simulink subsystem "Battery_Model"  (R2022a)
settings: Solver=VariableStepAuto  StartTime=0.0  StopTime=10.0  RelTol=1e-3
undefined symbols (not defined in the file): Battery, Np_Module
libraries: fl_lib x580, nesl_utility x386, ee_lib x96, simulink x96
(part 1 of 6)
settings Model: Creator=The MathWorks, Inc.  LastModifiedBy=The MathWorks, Inc.
settings SolverCC: MaxZcPerStep=1
settings DebuggingCC: UnconnectedInputMsg=warning  UnconnectedOutputMsg=warning  UnconnectedLineMsg=warning
settings RTWCC: DLArmComputeVersion=19.05

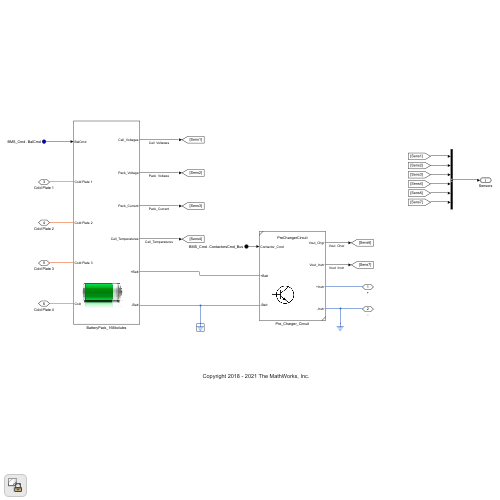
[thumbnail: Simulink's stored preview of the top-level diagram]
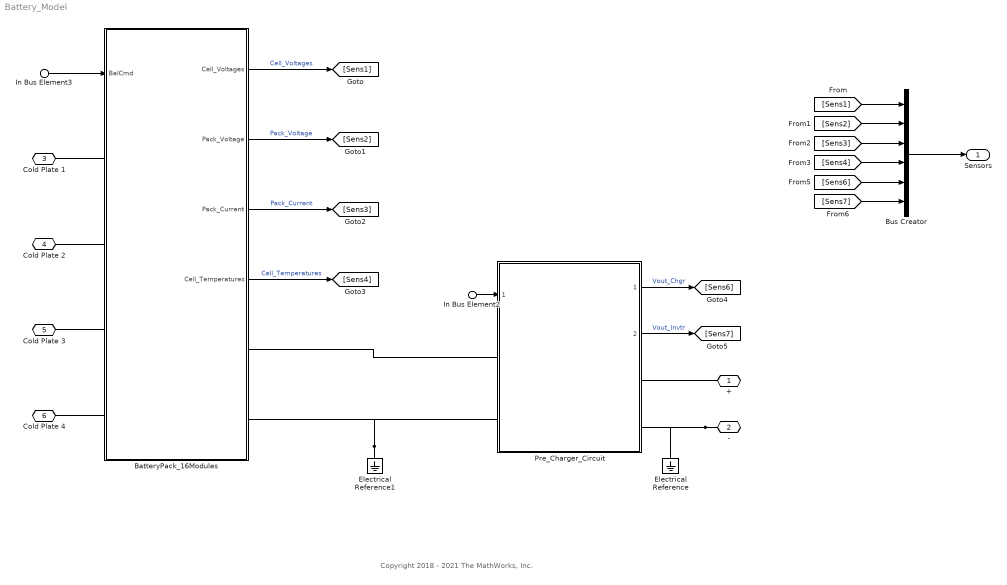
== system Battery_Model ==
  note: Copyright 2018 - 2021 The MathWorks, Inc.
  In Bus Element2 : Inport  PortName=BMS_Cmd  Element=ContactorsCmd_Bus
  In Bus Element3 : Inport  PortName=BMS_Cmd  Element=BalCmd
  BatteryPack_16Modules : Subsystem  VariantControl=NumModules == 16
      mask Display: image('Plant_Battery.jpg',[20,45,120,70])
  Bus Creator : BusCreator  Inputs=6  OutDataTypeStr=Bus: Sensors  NonVirtualBus=on
      settings: InheritFromInputs=off
  Electrical Reference : fl_lib/Electrical/Electrical Elements/Electrical Reference
      settings: SourceProductBaseCode=PW,SS,VE
  Electrical Reference1 : fl_lib/Electrical/Electrical Elements/Electrical Reference
      settings: SourceProductBaseCode=PW,SS,VE
  Pre_Charger_Circuit : Subsystem  ReferencedSubsystem=PreChangerCircuit
  + : PMIOPort  Side=Right
  - : PMIOPort  Port=2  Side=Right
  Cold Plate 1 : PMIOPort  Port=3  Side=Left
  Cold Plate 2 : PMIOPort  Port=4  Side=Left
  Cold Plate 3 : PMIOPort  Port=5  Side=Left
  Cold Plate 4 : PMIOPort  Port=6  Side=Left
  Sensors : Outport  OutDataTypeStr=Bus: Sensors  VectorParamsAs1DForOutWhenUnconnected=off  BusOutputAsStruct=on
  wires:
  [Sens6] -> Bus Creator/5
  Pre_Charger_Circuit/1 -> [Sens6]  "Vout_Chgr"
  [Sens3] -> Bus Creator/3
  In Bus Element2/1 -> Pre_Charger_Circuit/1
  [Sens7] -> Bus Creator/6
  [Sens1] -> Bus Creator/1
  [Sens2] -> Bus Creator/2
  [Sens4] -> Bus Creator/4
  Pre_Charger_Circuit/2 -> [Sens7]  "Vout_Invtr"
  BatteryPack_16Modules/1(Cell_Voltages) -> [Sens1]  "Cell_Voltages"
  Bus Creator/1 -> Sensors/1
  BatteryPack_16Modules/4(Cell_Temperatures) -> [Sens4]  "Cell_Temperatures"
  BatteryPack_16Modules/3(Pack_Current) -> [Sens3]  "Pack_Current"
  BatteryPack_16Modules/2(Pack_Voltage) -> [Sens2]  "Pack_Voltage"
  In Bus Element3/1 -> BatteryPack_16Modules/1(BalCmd)
  connections:
  -/RConn1 -- Electrical Reference/LConn1 -- Pre_Charger_Circuit/RConn2
  Electrical Reference1/LConn1 -- BatteryPack_16Modules/RConn2 -- Pre_Charger_Circuit/LConn2
  Pre_Charger_Circuit/RConn1 -- +/RConn1
  Pre_Charger_Circuit/LConn1 -- BatteryPack_16Modules/RConn1
  Cold Plate 1/RConn1 -- BatteryPack_16Modules/LConn1
  Cold Plate 2/RConn1 -- BatteryPack_16Modules/LConn2
  Cold Plate 3/RConn1 -- BatteryPack_16Modules/LConn3
  Cold Plate 4/RConn1 -- BatteryPack_16Modules/LConn4

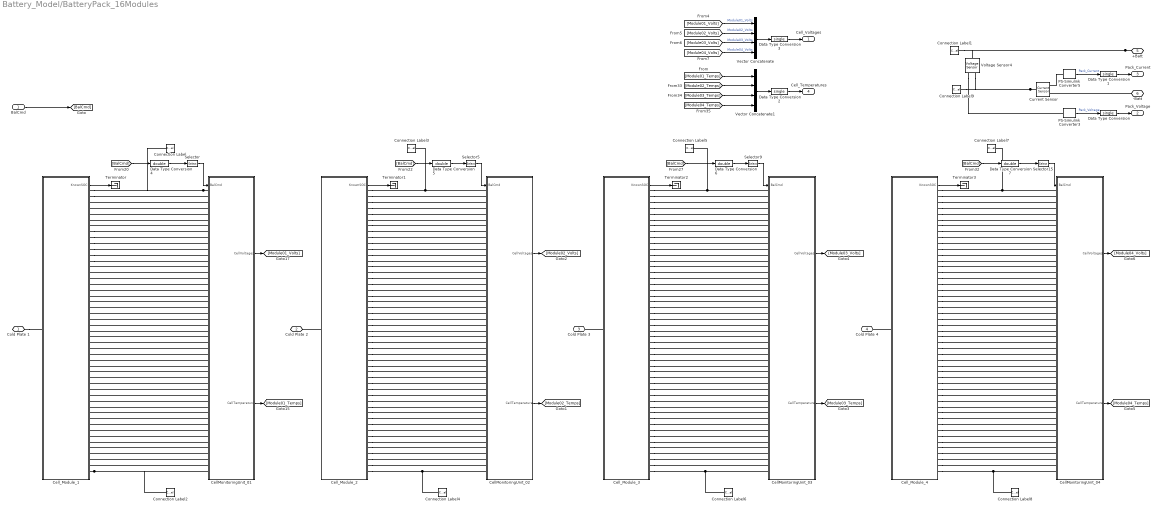
== system Battery_Model/BatteryPack_16Modules ==
  BalCmd : Inport
  CellMonitoringUnit_01 : Subsystem
  CellMonitoringUnit_02 : Subsystem
  CellMonitoringUnit_03 : Subsystem
  CellMonitoringUnit_04 : Subsystem
  Cell_Module_1 : Subsystem
  Cell_Module_2 : Subsystem
  Cell_Module_3 : Subsystem
  Cell_Module_4 : Subsystem
  Connection Label : ConnectionLabel  Label=BattPos
  Connection Label1 : ConnectionLabel  Label=BattPos
  Connection Label2 : ConnectionLabel  Label=BattA
  Connection Label3 : ConnectionLabel  Label=BattA
  Connection Label4 : ConnectionLabel  Label=BattB
  Connection Label5 : ConnectionLabel  Label=BattB
  Connection Label6 : ConnectionLabel  Label=BattC
  Connection Label7 : ConnectionLabel  Label=BattC
  Connection Label8 : ConnectionLabel  Label=BattNeg
  Connection Label9 : ConnectionLabel  Label=BattNeg
  Current Sensor : fl_lib/Electrical/Electrical Sensors/Current Sensor
      settings: SourceProductBaseCode=PW,SS,VE
  Data Type Conversion{,1..3} (4 alike) : DataTypeConversion  OutDataTypeStr=single  SaturateOnIntegerOverflow=off  RndMeth=Floor
  Data Type Conversion{4..7} (4 alike) : DataTypeConversion  OutDataTypeStr=double  SaturateOnIntegerOverflow=off  RndMeth=Floor
  PS-Simulink Converter3 : nesl_utility/PS-Simulink Converter  PhysicalDomain=network_engine_domain  SubClassName=ps_output  LeftPortType=input  RightPortType=output  PseudoPeriodic=off  Frequencies=[]  VectorFormat=1-D array  Unit=V  AffineConversion=off
      settings: SourceProductBaseCode=SS,PW,VE
  PS-Simulink Converter5 : nesl_utility/PS-Simulink Converter  PhysicalDomain=network_engine_domain  SubClassName=ps_output  LeftPortType=input  RightPortType=output  PseudoPeriodic=off  Frequencies=[]  VectorFormat=1-D array  Unit=A  AffineConversion=off
      settings: SourceProductBaseCode=SS,PW,VE
  Selector : Selector  InputPortWidth=96  IndexOptions=Starting index (dialog)  Indices=[1]  OutputSizes=24
  Selector15 : Selector  InputPortWidth=96  IndexOptions=Starting index (dialog)  Indices=73  OutputSizes=24
  Selector5 : Selector  InputPortWidth=96  IndexOptions=Starting index (dialog)  Indices=25  OutputSizes=24
  Selector9 : Selector  InputPortWidth=96  IndexOptions=Starting index (dialog)  Indices=49  OutputSizes=24
  Terminator{,1..3} (4 alike) : Terminator
  Vector Concatenate : Concatenate  NumInputs=4
  Vector Concatenate1 : Concatenate  NumInputs=4
  Voltage Sensor4 : fl_lib/Electrical/Electrical Sensors/Voltage Sensor
      settings: SourceProductBaseCode=PW,SS,VE
  Cold Plate 1 : PMIOPort  Side=Left
  Cold Plate 2 : PMIOPort  Port=2  Side=Left
  Cold Plate 3 : PMIOPort  Port=3  Side=Left
  Cold Plate 4 : PMIOPort  Port=4  Side=Left
  +Batt : PMIOPort  Port=5  Side=Right
  -Batt : PMIOPort  Port=6  Side=Right
  Cell_Voltages : Outport  VectorParamsAs1DForOutWhenUnconnected=off
  Pack_Voltage : Outport  Port=2  VectorParamsAs1DForOutWhenUnconnected=off
  Pack_Current : Outport  Port=3  VectorParamsAs1DForOutWhenUnconnected=off
  Cell_Temperatures : Outport  Port=4  VectorParamsAs1DForOutWhenUnconnected=off
  wires:
  Data Type Conversion7/1 -> Selector15/1
  Data Type Conversion6/1 -> Selector9/1
  Data Type Conversion5/1 -> Selector5/1
  Data Type Conversion4/1 -> Selector/1
  CellMonitoringUnit_04/2(CellTemperature) -> [Module04_Temps]
  Cell_Module_4/1(KnownSOC) -> Terminator3/1
  CellMonitoringUnit_04/1(CellVoltages) -> [Module04_Volts]
  Selector15/1 -> CellMonitoringUnit_04/1(BalCmd)
  CellMonitoringUnit_03/2(CellTemperature) -> [Module03_Temps]
  Cell_Module_3/1(KnownSOC) -> Terminator2/1
  CellMonitoringUnit_03/1(CellVoltages) -> [Module03_Volts]
  Selector9/1 -> CellMonitoringUnit_03/1(BalCmd)
  CellMonitoringUnit_02/2(CellTemperature) -> [Module02_Temps]
  Cell_Module_2/1(KnownSOC) -> Terminator1/1
  CellMonitoringUnit_02/1(CellVoltages) -> [Module02_Volts]
  Selector5/1 -> CellMonitoringUnit_02/1(BalCmd)
  Cell_Module_1/1(KnownSOC) -> Terminator/1
  Data Type Conversion3/1 -> Cell_Voltages/1
  Data Type Conversion2/1 -> Cell_Temperatures/1
  CellMonitoringUnit_01/1(CellVoltages) -> [Module01_Volts]
  CellMonitoringUnit_01/2(CellTemperature) -> [Module01_Temps]
  Vector Concatenate1/1 -> Data Type Conversion2/1
  [Module04_Temps] -> Vector Concatenate1/4
  [Module03_Temps] -> Vector Concatenate1/3
  [Module02_Temps] -> Vector Concatenate1/2
  [Module01_Temps] -> Vector Concatenate1/1
  Data Type Conversion1/1 -> Pack_Current/1
  Data Type Conversion/1 -> Pack_Voltage/1
  [BalCmd] -> Data Type Conversion7/1
  [BalCmd] -> Data Type Conversion6/1
  [BalCmd] -> Data Type Conversion5/1
  Selector/1 -> CellMonitoringUnit_01/1(BalCmd)
  [BalCmd] -> Data Type Conversion4/1
  [Module04_Volts] -> Vector Concatenate/4  "Module04_Volts"
  [Module03_Volts] -> Vector Concatenate/3  "Module03_Volts"
  [Module02_Volts] -> Vector Concatenate/2  "Module02_Volts"
  Vector Concatenate/1 -> Data Type Conversion3/1
  [Module01_Volts] -> Vector Concatenate/1  "Module01_Volts"
  PS-Simulink Converter5/1 -> Data Type Conversion1/1  "Pack_Current"
  PS-Simulink Converter3/1 -> Data Type Conversion/1  "Pack_Voltage"
  BalCmd/1 -> [BalCmd]
  connections:
  Cell_Module_4/RConn40 -- CellMonitoringUnit_04/LConn40
  Cell_Module_4/RConn10 -- CellMonitoringUnit_04/LConn10
  Cell_Module_4/RConn35 -- CellMonitoringUnit_04/LConn35
  Cell_Module_4/RConn24 -- CellMonitoringUnit_04/LConn24
  Cell_Module_4/RConn5 -- CellMonitoringUnit_04/LConn5
  Cell_Module_4/RConn44 -- CellMonitoringUnit_04/LConn44
  Cell_Module_4/RConn29 -- CellMonitoringUnit_04/LConn29
  Cell_Module_4/RConn33 -- CellMonitoringUnit_04/LConn33
  Cell_Module_4/RConn3 -- CellMonitoringUnit_04/LConn3
  Cell_Module_4/RConn9 -- CellMonitoringUnit_04/LConn9
  Cell_Module_4/RConn30 -- CellMonitoringUnit_04/LConn30
  Cell_Module_4/RConn18 -- CellMonitoringUnit_04/LConn18
  Cell_Module_4/RConn16 -- CellMonitoringUnit_04/LConn16
  Cell_Module_4/RConn19 -- CellMonitoringUnit_04/LConn19
  Cell_Module_4/RConn36 -- CellMonitoringUnit_04/LConn36
  Cell_Module_4/RConn46 -- CellMonitoringUnit_04/LConn46
  Cell_Module_4/RConn4 -- CellMonitoringUnit_04/LConn4
  Cell_Module_4/RConn47 -- CellMonitoringUnit_04/LConn47
  Cell_Module_4/RConn20 -- CellMonitoringUnit_04/LConn20
  Cell_Module_4/RConn42 -- CellMonitoringUnit_04/LConn42
  Cell_Module_4/RConn27 -- CellMonitoringUnit_04/LConn27
  Cell_Module_4/RConn32 -- CellMonitoringUnit_04/LConn32
  Cell_Module_4/RConn23 -- CellMonitoringUnit_04/LConn23
  Cell_Module_4/RConn15 -- CellMonitoringUnit_04/LConn15
  Cell_Module_4/RConn45 -- CellMonitoringUnit_04/LConn45
  Cell_Module_4/RConn17 -- CellMonitoringUnit_04/LConn17
  Cell_Module_4/RConn39 -- CellMonitoringUnit_04/LConn39
  Cell_Module_4/RConn12 -- CellMonitoringUnit_04/LConn12
  Cell_Module_4/RConn26 -- CellMonitoringUnit_04/LConn26
  Cell_Module_4/RConn6 -- CellMonitoringUnit_04/LConn6
  Cell_Module_4/RConn21 -- CellMonitoringUnit_04/LConn21
  Cell_Module_4/RConn48 -- CellMonitoringUnit_04/LConn48
  Cell_Module_4/RConn2 -- CellMonitoringUnit_04/LConn2
  Cell_Module_4/RConn31 -- CellMonitoringUnit_04/LConn31
  Cell_Module_4/RConn11 -- CellMonitoringUnit_04/LConn11
  Cell_Module_4/RConn38 -- CellMonitoringUnit_04/LConn38
  Cell_Module_4/RConn14 -- CellMonitoringUnit_04/LConn14
  Cell_Module_4/RConn8 -- CellMonitoringUnit_04/LConn8
  Cell_Module_4/RConn22 -- CellMonitoringUnit_04/LConn22
  Cell_Module_4/RConn13 -- CellMonitoringUnit_04/LConn13
  Cell_Module_4/RConn34 -- CellMonitoringUnit_04/LConn34
  Cell_Module_4/LConn1 -- Cold Plate 4/RConn1
  Cell_Module_4/RConn37 -- CellMonitoringUnit_04/LConn37
  Cell_Module_4/RConn43 -- CellMonitoringUnit_04/LConn43
  Cell_Module_4/RConn41 -- CellMonitoringUnit_04/LConn41
  Cell_Module_4/RConn7 -- CellMonitoringUnit_04/LConn7
  Cell_Module_4/RConn28 -- CellMonitoringUnit_04/LConn28
  Cell_Module_4/RConn25 -- CellMonitoringUnit_04/LConn25
  Cell_Module_4/RConn49 -- Connection Label8/LConn1 -- CellMonitoringUnit_04/LConn49
  Cell_Module_4/RConn1 -- Connection Label7/LConn1 -- CellMonitoringUnit_04/LConn1
  Cell_Module_3/RConn18 -- CellMonitoringUnit_03/LConn18
  Cell_Module_3/RConn10 -- CellMonitoringUnit_03/LConn10
  Cell_Module_3/RConn39 -- CellMonitoringUnit_03/LConn39
  Cell_Module_3/RConn44 -- CellMonitoringUnit_03/LConn44
  Cell_Module_3/RConn46 -- CellMonitoringUnit_03/LConn46
  Cell_Module_3/RConn24 -- CellMonitoringUnit_03/LConn24
  Cell_Module_3/RConn33 -- CellMonitoringUnit_03/LConn33
  Cell_Module_3/RConn32 -- CellMonitoringUnit_03/LConn32
  Cell_Module_3/RConn5 -- CellMonitoringUnit_03/LConn5
  Cell_Module_3/RConn17 -- CellMonitoringUnit_03/LConn17
  Cell_Module_3/RConn29 -- CellMonitoringUnit_03/LConn29
  Cell_Module_3/RConn9 -- CellMonitoringUnit_03/LConn9
  Cell_Module_3/RConn16 -- CellMonitoringUnit_03/LConn16
  Cell_Module_3/RConn48 -- CellMonitoringUnit_03/LConn48
  Cell_Module_3/RConn19 -- CellMonitoringUnit_03/LConn19
  Cell_Module_3/RConn36 -- CellMonitoringUnit_03/LConn36
  Cell_Module_3/RConn11 -- CellMonitoringUnit_03/LConn11
  Cell_Module_3/RConn4 -- CellMonitoringUnit_03/LConn4
  Cell_Module_3/RConn47 -- CellMonitoringUnit_03/LConn47
  Cell_Module_3/RConn20 -- CellMonitoringUnit_03/LConn20
  Cell_Module_3/RConn42 -- CellMonitoringUnit_03/LConn42
  Cell_Module_3/RConn21 -- CellMonitoringUnit_03/LConn21
  Cell_Module_3/RConn45 -- CellMonitoringUnit_03/LConn45
  Cell_Module_3/RConn15 -- CellMonitoringUnit_03/LConn15
  Cell_Module_3/RConn30 -- CellMonitoringUnit_03/LConn30
  Cell_Module_3/RConn31 -- CellMonitoringUnit_03/LConn31
  Cell_Module_3/RConn23 -- CellMonitoringUnit_03/LConn23
  Cell_Module_3/RConn40 -- CellMonitoringUnit_03/LConn40
  Cell_Module_3/RConn35 -- CellMonitoringUnit_03/LConn35
  Cell_Module_3/RConn12 -- CellMonitoringUnit_03/LConn12
  Cell_Module_3/RConn26 -- CellMonitoringUnit_03/LConn26
  Cell_Module_3/RConn6 -- CellMonitoringUnit_03/LConn6
  Cell_Module_3/RConn2 -- CellMonitoringUnit_03/LConn2
  Cell_Module_3/RConn38 -- CellMonitoringUnit_03/LConn38
  Cell_Module_3/RConn3 -- CellMonitoringUnit_03/LConn3
  Cell_Module_3/RConn8 -- CellMonitoringUnit_03/LConn8
  Cell_Module_3/RConn25 -- CellMonitoringUnit_03/LConn25
  Cell_Module_3/RConn22 -- CellMonitoringUnit_03/LConn22
  Cell_Module_3/RConn13 -- CellMonitoringUnit_03/LConn13
  Cell_Module_3/RConn14 -- CellMonitoringUnit_03/LConn14
  Cell_Module_3/RConn34 -- CellMonitoringUnit_03/LConn34
  Cell_Module_3/RConn37 -- CellMonitoringUnit_03/LConn37
  Cell_Module_3/RConn43 -- CellMonitoringUnit_03/LConn43
  Cell_Module_3/RConn41 -- CellMonitoringUnit_03/LConn41
  Cell_Module_3/LConn1 -- Cold Plate 3/RConn1
  Cell_Module_3/RConn7 -- CellMonitoringUnit_03/LConn7
  Cell_Module_3/RConn28 -- CellMonitoringUnit_03/LConn28
  Cell_Module_3/RConn27 -- CellMonitoringUnit_03/LConn27
  Cell_Module_3/RConn49 -- Connection Label6/LConn1 -- CellMonitoringUnit_03/LConn49
  Cell_Module_3/RConn1 -- Connection Label5/LConn1 -- CellMonitoringUnit_03/LConn1
  Cell_Module_2/RConn18 -- CellMonitoringUnit_02/LConn18
  Cell_Module_2/RConn10 -- CellMonitoringUnit_02/LConn10
  Cell_Module_2/RConn39 -- CellMonitoringUnit_02/LConn39
  Cell_Module_2/RConn44 -- CellMonitoringUnit_02/LConn44
  Cell_Module_2/RConn46 -- CellMonitoringUnit_02/LConn46
  Cell_Module_2/RConn24 -- CellMonitoringUnit_02/LConn24
  Cell_Module_2/RConn33 -- CellMonitoringUnit_02/LConn33
  Cell_Module_2/RConn32 -- CellMonitoringUnit_02/LConn32
  Cell_Module_2/RConn5 -- CellMonitoringUnit_02/LConn5
  Cell_Module_2/RConn17 -- CellMonitoringUnit_02/LConn17
  Cell_Module_2/RConn29 -- CellMonitoringUnit_02/LConn29
  Cell_Module_2/RConn9 -- CellMonitoringUnit_02/LConn9
  Cell_Module_2/RConn16 -- CellMonitoringUnit_02/LConn16
  Cell_Module_2/RConn48 -- CellMonitoringUnit_02/LConn48
  Cell_Module_2/RConn19 -- CellMonitoringUnit_02/LConn19
  Cell_Module_2/RConn36 -- CellMonitoringUnit_02/LConn36
  Cell_Module_2/RConn11 -- CellMonitoringUnit_02/LConn11
  Cell_Module_2/RConn4 -- CellMonitoringUnit_02/LConn4
  Cell_Module_2/RConn47 -- CellMonitoringUnit_02/LConn47
  Cell_Module_2/RConn20 -- CellMonitoringUnit_02/LConn20
  Cell_Module_2/RConn42 -- CellMonitoringUnit_02/LConn42
  Cell_Module_2/RConn21 -- CellMonitoringUnit_02/LConn21
  Cell_Module_2/RConn45 -- CellMonitoringUnit_02/LConn45
  Cell_Module_2/RConn15 -- CellMonitoringUnit_02/LConn15
  Cell_Module_2/RConn30 -- CellMonitoringUnit_02/LConn30
  Cell_Module_2/RConn31 -- CellMonitoringUnit_02/LConn31
  Cell_Module_2/RConn23 -- CellMonitoringUnit_02/LConn23
  Cell_Module_2/RConn40 -- CellMonitoringUnit_02/LConn40
  Cell_Module_2/RConn35 -- CellMonitoringUnit_02/LConn35
  Cell_Module_2/RConn12 -- CellMonitoringUnit_02/LConn12
  Cell_Module_2/RConn26 -- CellMonitoringUnit_02/LConn26
  Cell_Module_2/RConn6 -- CellMonitoringUnit_02/LConn6
  Cell_Module_2/RConn2 -- CellMonitoringUnit_02/LConn2
  Cell_Module_2/RConn38 -- CellMonitoringUnit_02/LConn38
  Cell_Module_2/RConn3 -- CellMonitoringUnit_02/LConn3
  Cell_Module_2/RConn8 -- CellMonitoringUnit_02/LConn8
  Cell_Module_2/RConn25 -- CellMonitoringUnit_02/LConn25
  Cell_Module_2/RConn22 -- CellMonitoringUnit_02/LConn22
  Cell_Module_2/RConn13 -- CellMonitoringUnit_02/LConn13
  Cell_Module_2/RConn14 -- CellMonitoringUnit_02/LConn14
  Cell_Module_2/RConn34 -- CellMonitoringUnit_02/LConn34
  Cell_Module_2/RConn37 -- CellMonitoringUnit_02/LConn37
  Cell_Module_2/RConn43 -- CellMonitoringUnit_02/LConn43
  Cell_Module_2/RConn41 -- CellMonitoringUnit_02/LConn41
  Cell_Module_2/LConn1 -- Cold Plate 2/RConn1
  Cell_Module_2/RConn7 -- CellMonitoringUnit_02/LConn7
  Cell_Module_2/RConn28 -- CellMonitoringUnit_02/LConn28
  Cell_Module_2/RConn27 -- CellMonitoringUnit_02/LConn27
  Cell_Module_2/RConn49 -- Connection Label4/LConn1 -- CellMonitoringUnit_02/LConn49
  Cell_Module_2/RConn1 -- Connection Label3/LConn1 -- CellMonitoringUnit_02/LConn1
  Cold Plate 1/RConn1 -- Cell_Module_1/LConn1
  CellMonitoringUnit_01/LConn48 -- Cell_Module_1/RConn48
  Cell_Module_1/RConn49 -- CellMonitoringUnit_01/LConn49 -- Connection Label2/LConn1
  CellMonitoringUnit_01/LConn47 -- Cell_Module_1/RConn47
  CellMonitoringUnit_01/LConn46 -- Cell_Module_1/RConn46
  CellMonitoringUnit_01/LConn45 -- Cell_Module_1/RConn45
  CellMonitoringUnit_01/LConn44 -- Cell_Module_1/RConn44
  CellMonitoringUnit_01/LConn43 -- Cell_Module_1/RConn43
  CellMonitoringUnit_01/LConn42 -- Cell_Module_1/RConn42
  CellMonitoringUnit_01/LConn41 -- Cell_Module_1/RConn41
  CellMonitoringUnit_01/LConn40 -- Cell_Module_1/RConn40
  CellMonitoringUnit_01/LConn39 -- Cell_Module_1/RConn39
  CellMonitoringUnit_01/LConn38 -- Cell_Module_1/RConn38
  CellMonitoringUnit_01/LConn37 -- Cell_Module_1/RConn37
  CellMonitoringUnit_01/LConn36 -- Cell_Module_1/RConn36
  CellMonitoringUnit_01/LConn35 -- Cell_Module_1/RConn35
  CellMonitoringUnit_01/LConn34 -- Cell_Module_1/RConn34
  CellMonitoringUnit_01/LConn33 -- Cell_Module_1/RConn33
  CellMonitoringUnit_01/LConn32 -- Cell_Module_1/RConn32
  CellMonitoringUnit_01/LConn31 -- Cell_Module_1/RConn31
  CellMonitoringUnit_01/LConn30 -- Cell_Module_1/RConn30
  CellMonitoringUnit_01/LConn29 -- Cell_Module_1/RConn29
  CellMonitoringUnit_01/LConn28 -- Cell_Module_1/RConn28
  CellMonitoringUnit_01/LConn27 -- Cell_Module_1/RConn27
  CellMonitoringUnit_01/LConn26 -- Cell_Module_1/RConn26
  CellMonitoringUnit_01/LConn25 -- Cell_Module_1/RConn25
  CellMonitoringUnit_01/LConn24 -- Cell_Module_1/RConn24
  CellMonitoringUnit_01/LConn23 -- Cell_Module_1/RConn23
  CellMonitoringUnit_01/LConn22 -- Cell_Module_1/RConn22
  CellMonitoringUnit_01/LConn21 -- Cell_Module_1/RConn21
  CellMonitoringUnit_01/LConn20 -- Cell_Module_1/RConn20
  CellMonitoringUnit_01/LConn19 -- Cell_Module_1/RConn19
  CellMonitoringUnit_01/LConn18 -- Cell_Module_1/RConn18
  CellMonitoringUnit_01/LConn17 -- Cell_Module_1/RConn17
  CellMonitoringUnit_01/LConn16 -- Cell_Module_1/RConn16
  CellMonitoringUnit_01/LConn15 -- Cell_Module_1/RConn15
  CellMonitoringUnit_01/LConn14 -- Cell_Module_1/RConn14
  Current Sensor/LConn1 -- Connection Label9/LConn1 -- Voltage Sensor4/RConn2
  +Batt/RConn1 -- Connection Label1/LConn1 -- Voltage Sensor4/LConn1
  Cell_Module_1/RConn13 -- CellMonitoringUnit_01/LConn13
  CellMonitoringUnit_01/LConn3 -- Cell_Module_1/RConn3
  CellMonitoringUnit_01/LConn4 -- Cell_Module_1/RConn4
  CellMonitoringUnit_01/LConn5 -- Cell_Module_1/RConn5
  CellMonitoringUnit_01/LConn6 -- Cell_Module_1/RConn6
  CellMonitoringUnit_01/LConn7 -- Cell_Module_1/RConn7
  Cell_Module_1/RConn8 -- CellMonitoringUnit_01/LConn8
  Cell_Module_1/RConn9 -- CellMonitoringUnit_01/LConn9
  Cell_Module_1/RConn10 -- CellMonitoringUnit_01/LConn10
  Cell_Module_1/RConn11 -- CellMonitoringUnit_01/LConn11
  Cell_Module_1/RConn12 -- CellMonitoringUnit_01/LConn12
  Cell_Module_1/RConn2 -- CellMonitoringUnit_01/LConn2
  PS-Simulink Converter5/LConn1 -- Current Sensor/RConn1
  Voltage Sensor4/RConn1 -- PS-Simulink Converter3/LConn1
  -Batt/RConn1 -- Current Sensor/RConn2
  CellMonitoringUnit_01/LConn1 -- Cell_Module_1/RConn1 -- Connection Label/LConn1

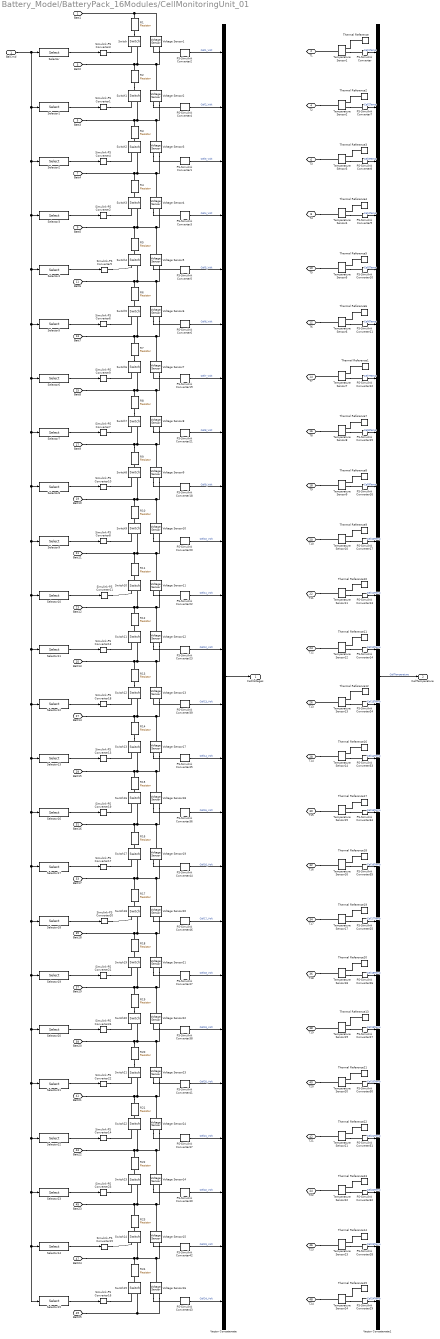
== system Battery_Model/BatteryPack_16Modules/CellMonitoringUnit_01 ==
  BalCmd : Inport
  PS-Simulink Converter{,7..17,24..35} (24 alike) : nesl_utility/PS-Simulink Converter  PhysicalDomain=network_engine_domain  SubClassName=ps_output  LeftPortType=input  RightPortType=output  PseudoPeriodic=off  Frequencies=[]  VectorFormat=1-D array  Unit=degC  AffineConversion=on
      settings: SourceProductBaseCode=SS,PW,VE
  PS-Simulink Converter{1..6,18..23,36..47} (24 alike) : nesl_utility/PS-Simulink Converter  PhysicalDomain=network_engine_domain  SubClassName=ps_output  LeftPortType=input  RightPortType=output  PseudoPeriodic=off  Frequencies=[]  VectorFormat=1-D array  Unit=V  AffineConversion=off
      settings: SourceProductBaseCode=SS,PW,VE
  R{1..24} (24 alike) : fl_lib/Electrical/Electrical Elements/Resistor  R=Battery.R_bleed Ohm  i_specify=off  i_priority=None  i=0 A  i_nominal_specify=off  i_nominal_unit=A  i_nominal_value=1  v_specify=off  v_priority=None  v=0 V  v_nominal_specify=off  v_nominal_unit=V  v_nominal_value=1
      R1 settings: SourceProductBaseCode=PW,SS,VE  LogSimulationData=on
      R10 settings: SourceProductBaseCode=PW,SS,VE
      R11 settings: SourceProductBaseCode=PW,SS,VE
      R12 settings: SourceProductBaseCode=PW,SS,VE
      R13 settings: SourceProductBaseCode=PW,SS,VE  LogSimulationData=on
      R14 settings: SourceProductBaseCode=PW,SS,VE
      R15 settings: SourceProductBaseCode=PW,SS,VE
      R16 settings: SourceProductBaseCode=PW,SS,VE
      R17 settings: SourceProductBaseCode=PW,SS,VE
      R18 settings: SourceProductBaseCode=PW,SS,VE
      R19 settings: SourceProductBaseCode=PW,SS,VE  LogSimulationData=on
      R2 settings: SourceProductBaseCode=PW,SS,VE
      R20 settings: SourceProductBaseCode=PW,SS,VE
      R21 settings: SourceProductBaseCode=PW,SS,VE
      R22 settings: SourceProductBaseCode=PW,SS,VE
      R23 settings: SourceProductBaseCode=PW,SS,VE
      R24 settings: SourceProductBaseCode=PW,SS,VE
      R3 settings: SourceProductBaseCode=PW,SS,VE
      R4 settings: SourceProductBaseCode=PW,SS,VE
      R5 settings: SourceProductBaseCode=PW,SS,VE
      R6 settings: SourceProductBaseCode=PW,SS,VE
      R7 settings: SourceProductBaseCode=PW,SS,VE  LogSimulationData=on
      R8 settings: SourceProductBaseCode=PW,SS,VE
      R9 settings: SourceProductBaseCode=PW,SS,VE
  Selector : Selector  IndexOptions=Index vector (dialog)  Indices=1  OutputSizes=1
  Selector1 : Selector  IndexOptions=Index vector (dialog)  Indices=2  OutputSizes=1
  Selector10 : Selector  IndexOptions=Index vector (dialog)  Indices=11  OutputSizes=1
  Selector11 : Selector  IndexOptions=Index vector (dialog)  Indices=12  OutputSizes=1
  Selector12 : Selector  IndexOptions=Index vector (dialog)  Indices=13  OutputSizes=1
  Selector13 : Selector  IndexOptions=Index vector (dialog)  Indices=14  OutputSizes=1
  Selector14 : Selector  IndexOptions=Index vector (dialog)  Indices=23  OutputSizes=1
  Selector15 : Selector  IndexOptions=Index vector (dialog)  Indices=24  OutputSizes=1
  Selector16 : Selector  IndexOptions=Index vector (dialog)  Indices=15  OutputSizes=1
  Selector17 : Selector  IndexOptions=Index vector (dialog)  Indices=16  OutputSizes=1
  Selector18 : Selector  IndexOptions=Index vector (dialog)  Indices=17  OutputSizes=1
  Selector19 : Selector  IndexOptions=Index vector (dialog)  Indices=18  OutputSizes=1
  Selector2 : Selector  IndexOptions=Index vector (dialog)  Indices=3  OutputSizes=1
  Selector20 : Selector  IndexOptions=Index vector (dialog)  Indices=19  OutputSizes=1
  Selector21 : Selector  IndexOptions=Index vector (dialog)  Indices=20  OutputSizes=1
  Selector22 : Selector  IndexOptions=Index vector (dialog)  Indices=21  OutputSizes=1
  Selector23 : Selector  IndexOptions=Index vector (dialog)  Indices=22  OutputSizes=1
  Selector3 : Selector  IndexOptions=Index vector (dialog)  Indices=4  OutputSizes=1
  Selector4 : Selector  IndexOptions=Index vector (dialog)  Indices=5  OutputSizes=1
  Selector5 : Selector  IndexOptions=Index vector (dialog)  Indices=6  OutputSizes=1
  Selector6 : Selector  IndexOptions=Index vector (dialog)  Indices=7  OutputSizes=1
  Selector7 : Selector  IndexOptions=Index vector (dialog)  Indices=8  OutputSizes=1
  Selector8 : Selector  IndexOptions=Index vector (dialog)  Indices=9  OutputSizes=1
  Selector9 : Selector  IndexOptions=Index vector (dialog)  Indices=10  OutputSizes=1
  Simulink-PS Converter{1..24} (24 alike) : nesl_utility/Simulink-PS Converter  PhysicalDomain=network_engine_domain  SubClassName=ps_input  LeftPortType=input  RightPortType=output  PseudoPeriodic=off  Frequencies=[]  NoiseDistribution=none  NoiseParameters=[]  Unit=1  AffineConversion=off  FilteringAndDerivatives=zero  SimscapeFilterOrder=1  InputFilterTimeConstant=0.001  UdotUserProvided=1
      settings: SourceProductBaseCode=SS,PW,VE
  Switch{,1..23} (24 alike) : fl_lib/Electrical/Electrical Elements/Switch  R_closed=0.01 Ohm  G_open=1e-8 1/Ohm  Threshold=0  i_specify=off  i_priority=None  i=0 A  i_nominal_specify=off  i_nominal_unit=A  i_nominal_value=1  v_specify=off  v_priority=None  v=0 V  v_nominal_specify=off  v_nominal_unit=V  v_nominal_value=1
      settings: SourceProductBaseCode=PW,SS,VE
  Temperature Sensor{1..24} (24 alike) : fl_lib/Thermal/Thermal Sensors/Temperature Sensor
      settings: SourceProductBaseCode=PW,SS,VE
  Thermal Reference{,1..23} (24 alike) : fl_lib/Thermal/Thermal Elements/Thermal Reference
      settings: SourceProductBaseCode=PW,SS,VE
  Vector Concatenate : Concatenate  NumInputs=24
  Vector Concatenate1 : Concatenate  NumInputs=24
  Voltage Sensor{1..24} (24 alike) : fl_lib/Electrical/Electrical Sensors/Voltage Sensor
      settings: SourceProductBaseCode=PW,SS,VE
  Batt1 : PMIOPort  Side=Left
  T1 : PMIOPort  Port=2  Side=Left
  Batt2 : PMIOPort  Port=3  Side=Left
  T2 : PMIOPort  Port=4  Side=Left
  Batt3 : PMIOPort  Port=5  Side=Left
  T3 : PMIOPort  Port=6  Side=Left
  Batt4 : PMIOPort  Port=7  Side=Left
  T4 : PMIOPort  Port=8  Side=Left
  Batt5 : PMIOPort  Port=9  Side=Left
  T5 : PMIOPort  Port=10  Side=Left
  Batt6 : PMIOPort  Port=11  Side=Left
  T6 : PMIOPort  Port=12  Side=Left
  Batt7 : PMIOPort  Port=13  Side=Left
  T7 : PMIOPort  Port=14  Side=Left
  Batt8 : PMIOPort  Port=15  Side=Left
  T8 : PMIOPort  Port=16  Side=Left
  Batt9 : PMIOPort  Port=17  Side=Left
  T9 : PMIOPort  Port=18  Side=Left
  Batt10 : PMIOPort  Port=19  Side=Left
  T10 : PMIOPort  Port=20  Side=Left
  Batt11 : PMIOPort  Port=21  Side=Left
  T11 : PMIOPort  Port=22  Side=Left
  Batt12 : PMIOPort  Port=23  Side=Left
  T12 : PMIOPort  Port=24  Side=Left
  Batt13 : PMIOPort  Port=25  Side=Left
  T13 : PMIOPort  Port=26  Side=Left
  Batt14 : PMIOPort  Port=27  Side=Left
  T14 : PMIOPort  Port=28  Side=Left
  Batt15 : PMIOPort  Port=29  Side=Left
  T15 : PMIOPort  Port=30  Side=Left
  Batt16 : PMIOPort  Port=31  Side=Left
  T16 : PMIOPort  Port=32  Side=Left
  Batt17 : PMIOPort  Port=33  Side=Left
  T17 : PMIOPort  Port=34  Side=Left
  Batt18 : PMIOPort  Port=35  Side=Left
  T18 : PMIOPort  Port=36  Side=Left
  Batt19 : PMIOPort  Port=37  Side=Left
  T19 : PMIOPort  Port=38  Side=Left
  Batt20 : PMIOPort  Port=39  Side=Left
  T20 : PMIOPort  Port=40  Side=Left
  Batt21 : PMIOPort  Port=41  Side=Left
  T21 : PMIOPort  Port=42  Side=Left
  Batt22 : PMIOPort  Port=43  Side=Left
  T22 : PMIOPort  Port=44  Side=Left
  Batt23 : PMIOPort  Port=45  Side=Left
  T23 : PMIOPort  Port=46  Side=Left
  Batt24 : PMIOPort  Port=47  Side=Left
  T24 : PMIOPort  Port=48  Side=Left
  Batt25 : PMIOPort  Port=49  Side=Left
  CellVoltages : Outport  VectorParamsAs1DForOutWhenUnconnected=off
  CellTemperature : Outport  Port=2  VectorParamsAs1DForOutWhenUnconnected=off
  wires:
  PS-Simulink Converter39/1 -> Vector Concatenate/13  "Cell13_Volt"
  Selector18/1 -> Simulink-PS Converter20/1
  PS-Simulink Converter45/1 -> Vector Concatenate/14  "Cell14_Volt"
  Selector23/1 -> Simulink-PS Converter23/1
  PS-Simulink Converter47/1 -> Vector Concatenate/18  "Cell18_Volt"
  PS-Simulink Converter40/1 -> Vector Concatenate/22  "Cell22_Volt"
  PS-Simulink Converter46/1 -> Vector Concatenate/17  "Cell17_Volt"
  Selector16/1 -> Simulink-PS Converter19/1
  PS-Simulink Converter42/1 -> Vector Concatenate/23  "Cell23_Volt"
  Selector21/1 -> Simulink-PS Converter22/1
  Selector14/1 -> Simulink-PS Converter15/1
  Selector22/1 -> Simulink-PS Converter14/1
  Selector20/1 -> Simulink-PS Converter24/1
  Selector15/1 -> Simulink-PS Converter16/1
  PS-Simulink Converter43/1 -> Vector Concatenate/24  "Cell24_Volt"
  PS-Simulink Converter41/1 -> Vector Concatenate/20  "Cell20_Volt"
  PS-Simulink Converter38/1 -> Vector Concatenate/19  "Cell19_Volt"
  PS-Simulink Converter37/1 -> Vector Concatenate/21  "Cell21_Volt"
  BalCmd/1 -> Selector3/1, Selector5/1, Selector9/1, Selector11/1, Selector12/1, Selector17/1, Selector19/1, Selector23/1, Selector15/1, Selector14/1, Selector22/1, Selector21/1, Selector20/1, Selector18/1, Selector16/1, Selector13/1, Selector10/1, Selector8/1, Selector7/1, Selector6/1, Selector4/1, Selector2/1, Selector1/1, Selector/1
  Selector13/1 -> Simulink-PS Converter13/1
  PS-Simulink Converter36/1 -> Vector Concatenate/15  "Cell15_Volt"
  Selector12/1 -> Simulink-PS Converter18/1
  Selector19/1 -> Simulink-PS Converter21/1
  Selector17/1 -> Simulink-PS Converter17/1
  PS-Simulink Converter44/1 -> Vector Concatenate/16  "Cell16_Volt"
  PS-Simulink Converter32/1 -> Vector Concatenate1/22  "Cell22Temp"
  PS-Simulink Converter35/1 -> Vector Concatenate1/16  "Cell16Temp"
  PS-Simulink Converter34/1 -> Vector Concatenate1/15  "Cell15Temp"
  PS-Simulink Converter26/1 -> Vector Concatenate1/18  "Cell18Temp"
  PS-Simulink Converter27/1 -> Vector Concatenate1/19  "Cell19Temp"
  PS-Simulink Converter29/1 -> Vector Concatenate1/24  "Cell24Temp"
  PS-Simulink Converter28/1 -> Vector Concatenate1/23  "Cell23Temp"
  PS-Simulink Converter31/1 -> Vector Concatenate1/21  "Cell21Temp"
  PS-Simulink Converter30/1 -> Vector Concatenate1/20  "Cell20Temp"
  PS-Simulink Converter25/1 -> Vector Concatenate1/17  "Cell17Temp"
  PS-Simulink Converter33/1 -> Vector Concatenate1/14  "Cell14Temp"
  PS-Simulink Converter24/1 -> Vector Concatenate1/13  "Cell13Temp"
  Selector10/1 -> Simulink-PS Converter11/1
  PS-Simulink Converter21/1 -> Vector Concatenate/8  "Cell8_Volt"
  PS-Simulink Converter19/1 -> Vector Concatenate/7  "Cell7_Volt"
  PS-Simulink Converter23/1 -> Vector Concatenate/12  "Cell12_Volt"
  PS-Simulink Converter22/1 -> Vector Concatenate/11  "Cell11_Volt"
  Selector7/1 -> Simulink-PS Converter7/1
  Selector8/1 -> Simulink-PS Converter10/1
  PS-Simulink Converter18/1 -> Vector Concatenate/9  "Cell9_Volt"
  Selector6/1 -> Simulink-PS Converter9/1
  Selector11/1 -> Simulink-PS Converter12/1
  Selector9/1 -> Simulink-PS Converter8/1
  PS-Simulink Converter20/1 -> Vector Concatenate/10  "Cell10_Volt"
  PS-Simulink Converter14/1 -> Vector Concatenate1/12  "Cell12Temp"
  PS-Simulink Converter16/1 -> Vector Concatenate1/9  "Cell9Temp"
  PS-Simulink Converter17/1 -> Vector Concatenate1/10  "Cell10Temp"
  PS-Simulink Converter13/1 -> Vector Concatenate1/11  "Cell11Temp"
  PS-Simulink Converter15/1 -> Vector Concatenate1/8  "Cell8Temp"
  PS-Simulink Converter12/1 -> Vector Concatenate1/7  "Cell7Temp"
  Vector Concatenate/1 -> CellVoltages/1
  Selector2/1 -> Simulink-PS Converter4/1
  Selector1/1 -> Simulink-PS Converter1/1
  Selector/1 -> Simulink-PS Converter3/1
  Selector3/1 -> Simulink-PS Converter2/1
  Selector4/1 -> Simulink-PS Converter5/1
  Selector5/1 -> Simulink-PS Converter6/1
  PS-Simulink Converter2/1 -> Vector Concatenate/1  "Cell1_Volt"
  PS-Simulink Converter4/1 -> Vector Concatenate/2  "Cell2_Volt"
  PS-Simulink Converter1/1 -> Vector Concatenate/3  "Cell3_Volt"
  PS-Simulink Converter3/1 -> Vector Concatenate/4  "Cell4_Volt"
  PS-Simulink Converter5/1 -> Vector Concatenate/5  "Cell5_Volt"
  PS-Simulink Converter6/1 -> Vector Concatenate/6  "Cell6_Volt"
  Vector Concatenate1/1 -> CellTemperature/1  "CellTemperature"
  PS-Simulink Converter/1 -> Vector Concatenate1/1  "Cell1Temp"
  PS-Simulink Converter9/1 -> Vector Concatenate1/4  "Cell4Temp"
  PS-Simulink Converter7/1 -> Vector Concatenate1/2  "Cell2Temp"
  PS-Simulink Converter8/1 -> Vector Concatenate1/3  "Cell3Temp"
  PS-Simulink Converter10/1 -> Vector Concatenate1/5  "Cell5Temp"
  PS-Simulink Converter11/1 -> Vector Concatenate1/6  "Cell6Temp"
  connections:
  Voltage Sensor24/RConn1 -- PS-Simulink Converter37/LConn1
  Simulink-PS Converter17/RConn1 -- Switch17/RConn1
  R20/RConn1 -- Switch21/LConn1
  R23/RConn1 -- Switch14/LConn1
  Simulink-PS Converter14/RConn1 -- Switch22/RConn1
  Simulink-PS Converter16/RConn1 -- Switch15/RConn1
  Simulink-PS Converter21/RConn1 -- Switch19/RConn1
  Voltage Sensor15/RConn1 -- PS-Simulink Converter42/LConn1
  R17/RConn1 -- Switch18/LConn1
  Simulink-PS Converter22/RConn1 -- Switch21/RConn1
  Simulink-PS Converter20/RConn1 -- Switch18/RConn1
  Switch19/LConn1 -- R18/RConn1
  Switch23/LConn1 -- R22/RConn1
  R19/RConn1 -- Switch20/LConn1
  Voltage Sensor16/RConn1 -- PS-Simulink Converter43/LConn1
  Voltage Sensor20/RConn1 -- PS-Simulink Converter46/LConn1
  Voltage Sensor14/RConn1 -- PS-Simulink Converter40/LConn1
  R15/RConn1 -- Switch16/LConn1
  R21/RConn1 -- Switch22/LConn1
  Switch17/LConn1 -- R16/RConn1
  Simulink-PS Converter13/RConn1 -- Switch13/RConn1
  Simulink-PS Converter18/RConn1 -- Switch12/RConn1
  Simulink-PS Converter24/RConn1 -- Switch20/RConn1
  PS-Simulink Converter38/LConn1 -- Voltage Sensor22/RConn1
  R13/RConn1 -- Switch12/LConn1
  Switch15/LConn1 -- R24/RConn1
  Voltage Sensor17/RConn1 -- PS-Simulink Converter45/LConn1
  Voltage Sensor18/RConn1 -- PS-Simulink Converter36/LConn1
  Voltage Sensor23/RConn1 -- PS-Simulink Converter41/LConn1
  Simulink-PS Converter23/RConn1 -- Switch23/RConn1
  Voltage Sensor19/RConn1 -- PS-Simulink Converter44/LConn1
  PS-Simulink Converter39/LConn1 -- Voltage Sensor13/RConn1
  R14/RConn1 -- Switch13/LConn1
  Voltage Sensor21/RConn1 -- PS-Simulink Converter47/LConn1
  Simulink-PS Converter15/RConn1 -- Switch14/RConn1
  Simulink-PS Converter19/RConn1 -- Switch16/RConn1
  Voltage Sensor16/RConn2 -- Switch15/RConn2 -- Batt25/RConn1
  R20/LConn1 -- Voltage Sensor23/LConn1 -- Voltage Sensor22/RConn2 -- Switch20/RConn2 -- Batt20/RConn1
  Voltage Sensor22/LConn1 -- Voltage Sensor21/RConn2 -- Switch19/RConn2 -- Batt19/RConn1 -- R19/LConn1
  Voltage Sensor17/RConn2 -- Batt15/RConn1 -- R15/LConn1 -- Switch13/RConn2 -- Voltage Sensor18/LConn1
  Batt17/RConn1 -- R17/LConn1 -- Voltage Sensor20/LConn1 -- Voltage Sensor19/RConn2 -- Switch17/RConn2
  Voltage Sensor17/LConn1 -- Voltage Sensor13/RConn2 -- Switch12/RConn2 -- Batt14/RConn1 -- R14/LConn1
  Switch23/RConn2 -- R23/LConn1 -- Batt23/RConn1 -- Voltage Sensor15/LConn1 -- Voltage Sensor14/RConn2
  R21/LConn1 -- Batt21/RConn1 -- Switch21/RConn2 -- Voltage Sensor23/RConn2 -- Voltage Sensor24/LConn1
  Voltage Sensor15/RConn2 -- Switch14/RConn2 -- Batt24/RConn1 -- R24/LConn1 -- Voltage Sensor16/LConn1
  Voltage Sensor18/RConn2 -- Batt16/RConn1 -- R16/LConn1 -- Switch16/RConn2 -- Voltage Sensor19/LConn1
  Voltage Sensor20/RConn2 -- Switch18/RConn2 -- Batt18/RConn1 -- R18/LConn1 -- Voltage Sensor21/LConn1
  Batt22/RConn1 -- R22/LConn1 -- Switch22/RConn2 -- Voltage Sensor14/LConn1 -- Voltage Sensor24/RConn2
  Temperature Sensor22/RConn2 -- PS-Simulink Converter32/LConn1
  Temperature Sensor20/RConn2 -- PS-Simulink Converter30/LConn1
  Thermal Reference21/LConn1 -- Temperature Sensor20/RConn1
  Temperature Sensor14/RConn2 -- PS-Simulink Converter33/LConn1
  Temperature Sensor19/RConn2 -- PS-Simulink Converter27/LConn1
  Temperature Sensor23/RConn2 -- PS-Simulink Converter28/LConn1
  Temperature Sensor19/LConn1 -- T19/RConn1
  T24/RConn1 -- Temperature Sensor24/LConn1
  T23/RConn1 -- Temperature Sensor23/LConn1
  T15/RConn1 -- Temperature Sensor15/LConn1
  T18/RConn1 -- Temperature Sensor18/LConn1
  T21/RConn1 -- Temperature Sensor21/LConn1
  Thermal Reference22/LConn1 -- Temperature Sensor21/RConn1
  Temperature Sensor24/RConn2 -- PS-Simulink Converter29/LConn1
  Temperature Sensor13/RConn2 -- PS-Simulink Converter24/LConn1
  Thermal Reference23/LConn1 -- Temperature Sensor22/RConn1
  T22/RConn1 -- Temperature Sensor22/LConn1
  T14/RConn1 -- Temperature Sensor14/LConn1
  Temperature Sensor18/RConn2 -- PS-Simulink Converter26/LConn1
  Thermal Reference12/LConn1 -- Temperature Sensor13/RConn1
  Thermal Reference15/LConn1 -- Temperature Sensor24/RConn1
  Thermal Reference14/LConn1 -- Temperature Sensor23/RConn1
  Thermal Reference13/LConn1 -- Temperature Sensor19/RConn1
  Temperature Sensor21/RConn2 -- PS-Simulink Converter31/LConn1
  Thermal Reference17/LConn1 -- Temperature Sensor15/RConn1
  Temperature Sensor15/RConn2 -- PS-Simulink Converter34/LConn1
  T20/RConn1 -- Temperature Sensor20/LConn1
  Thermal Reference16/LConn1 -- Temperature Sensor14/RConn1
  Temperature Sensor16/RConn2 -- PS-Simulink Converter35/LConn1
  Temperature Sensor17/RConn2 -- PS-Simulink Converter25/LConn1
  Temperature Sensor13/LConn1 -- T13/RConn1
  T17/RConn1 -- Temperature Sensor17/LConn1
  Thermal Reference19/LConn1 -- Temperature Sensor17/RConn1
  Thermal Reference18/LConn1 -- Temperature Sensor16/RConn1
  T16/RConn1 -- Temperature Sensor16/LConn1
  Thermal Reference20/LConn1 -- Temperature Sensor18/RConn1
  Simulink-PS Converter10/RConn1 -- Switch8/RConn1
  Switch11/LConn1 -- R12/RConn1
  Simulink-PS Converter12/RConn1 -- Switch11/RConn1
  R11/RConn1 -- Switch10/LConn1
  Simulink-PS Converter11/RConn1 -- Switch10/RConn1
  Simulink-PS Converter8/RConn1 -- Switch9/RConn1
  Voltage Sensor11/RConn1 -- PS-Simulink Converter22/LConn1
  R9/RConn1 -- Switch8/LConn1
  PS-Simulink Converter19/LConn1 -- Voltage Sensor7/RConn1
  Simulink-PS Converter9/RConn1 -- Switch6/RConn1
  Voltage Sensor9/RConn1 -- PS-Simulink Converter18/LConn1
  Voltage Sensor8/RConn1 -- PS-Simulink Converter21/LConn1
  R8/RConn1 -- Switch7/LConn1
  Voltage Sensor10/RConn1 -- PS-Simulink Converter20/LConn1
  Voltage Sensor12/RConn1 -- PS-Simulink Converter23/LConn1
  R7/RConn1 -- Switch6/LConn1
  Simulink-PS Converter7/RConn1 -- Switch7/RConn1
  Switch9/LConn1 -- R10/RConn1
  Voltage Sensor13/LConn1 -- Voltage Sensor12/RConn2 -- Switch11/RConn2 -- Batt13/RConn1 -- R13/LConn1
  R9/LConn1 -- Batt9/RConn1 -- Switch7/RConn2 -- Voltage Sensor8/RConn2 -- Voltage Sensor9/LConn1
  Batt11/RConn1 -- R11/LConn1 -- Voltage Sensor11/LConn1 -- Voltage Sensor10/RConn2 -- Switch9/RConn2
  Voltage Sensor11/RConn2 -- Switch10/RConn2 -- Batt12/RConn1 -- R12/LConn1 -- Voltage Sensor12/LConn1
  Voltage Sensor8/LConn1 -- Voltage Sensor7/RConn2 -- Switch6/RConn2 -- Batt8/RConn1 -- R8/LConn1
  Batt10/RConn1 -- R10/LConn1 -- Switch8/RConn2 -- Voltage Sensor10/LConn1 -- Voltage Sensor9/RConn2
  Thermal Reference8/LConn1 -- Temperature Sensor9/RConn1
  Temperature Sensor7/RConn2 -- PS-Simulink Converter12/LConn1
  T12/RConn1 -- Temperature Sensor12/LConn1
  Thermal Reference7/LConn1 -- Temperature Sensor8/RConn1
  T11/RConn1 -- Temperature Sensor11/LConn1
  T9/RConn1 -- Temperature Sensor9/LConn1
  Temperature Sensor7/LConn1 -- T7/RConn1
  T8/RConn1 -- Temperature Sensor8/LConn1
  Thermal Reference1/LConn1 -- Temperature Sensor7/RConn1
  Temperature Sensor12/RConn2 -- PS-Simulink Converter14/LConn1
  Thermal Reference10/LConn1 -- Temperature Sensor11/RConn1
  T10/RConn1 -- Temperature Sensor10/LConn1
  Thermal Reference11/LConn1 -- Temperature Sensor12/RConn1
  Temperature Sensor10/RConn2 -- PS-Simulink Converter17/LConn1
  Temperature Sensor9/RConn2 -- PS-Simulink Converter16/LConn1
  Thermal Reference9/LConn1 -- Temperature Sensor10/RConn1
  Temperature Sensor11/RConn2 -- PS-Simulink Converter13/LConn1
  Temperature Sensor8/RConn2 -- PS-Simulink Converter15/LConn1
  Voltage Sensor4/LConn1 -- Voltage Sensor3/RConn2 -- Batt4/RConn1 -- R4/LConn1 -- Switch2/RConn2
  Voltage Sensor3/RConn1 -- PS-Simulink Converter1/LConn1
  Simulink-PS Converter4/RConn1 -- Switch2/RConn1
  Simulink-PS Converter1/RConn1 -- Switch1/RConn1
  Simulink-PS Converter3/RConn1 -- Switch/RConn1
  R2/RConn1 -- Switch1/LConn1
  Voltage Sensor2/RConn1 -- PS-Simulink Converter4/LConn1
  PS-Simulink Converter2/LConn1 -- Voltage Sensor1/RConn1
  Batt1/RConn1 -- Voltage Sensor1/LConn1 -- R1/LConn1
  R3/RConn1 -- Switch2/LConn1
  R1/RConn1 -- Switch/LConn1
  Batt2/RConn1 -- Voltage Sensor2/LConn1 -- Voltage Sensor1/RConn2 -- Switch/RConn2 -- R2/LConn1
  Voltage Sensor3/LConn1 -- Batt3/RConn1 -- R3/LConn1 -- Switch1/RConn2 -- Voltage Sensor2/RConn2
  Voltage Sensor4/RConn2 -- Voltage Sensor5/LConn1 -- Switch3/RConn2 -- R5/LConn1 -- Batt5/RConn1
  Switch3/LConn1 -- R4/RConn1
  Simulink-PS Converter2/RConn1 -- Switch3/RConn1
  Switch4/RConn2 -- Batt6/RConn1 -- R6/LConn1 -- Voltage Sensor6/LConn1 -- Voltage Sensor5/RConn2
  Simulink-PS Converter5/RConn1 -- Switch4/RConn1
  R5/RConn1 -- Switch4/LConn1
  Voltage Sensor7/LConn1 -- Voltage Sensor6/RConn2 -- Switch5/RConn2 -- Batt7/RConn1 -- R7/LConn1
  Simulink-PS Converter6/RConn1 -- Switch5/RConn1
  Switch5/LConn1 -- R6/RConn1
  Voltage Sensor4/RConn1 -- PS-Simulink Converter3/LConn1
  Voltage Sensor5/RConn1 -- PS-Simulink Converter5/LConn1
  Voltage Sensor6/RConn1 -- PS-Simulink Converter6/LConn1
  Temperature Sensor3/RConn2 -- PS-Simulink Converter8/LConn1
  Temperature Sensor1/RConn2 -- PS-Simulink Converter/LConn1
  Temperature Sensor6/RConn2 -- PS-Simulink Converter11/LConn1
  Temperature Sensor4/RConn2 -- PS-Simulink Converter9/LConn1
  Thermal Reference3/LConn1 -- Temperature Sensor3/RConn1
  Temperature Sensor5/RConn2 -- PS-Simulink Converter10/LConn1
  Thermal Reference4/LConn1 -- Temperature Sensor4/RConn1
  Temperature Sensor2/RConn2 -- PS-Simulink Converter7/LConn1
  Thermal Reference6/LConn1 -- Temperature Sensor6/RConn1
  Thermal Reference2/LConn1 -- Temperature Sensor2/RConn1
  Thermal Reference5/LConn1 -- Temperature Sensor5/RConn1
  Temperature Sensor1/LConn1 -- T1/RConn1
  T2/RConn1 -- Temperature Sensor2/LConn1
  T3/RConn1 -- Temperature Sensor3/LConn1
  T4/RConn1 -- Temperature Sensor4/LConn1
  T5/RConn1 -- Temperature Sensor5/LConn1
  T6/RConn1 -- Temperature Sensor6/LConn1
  Thermal Reference/LConn1 -- Temperature Sensor1/RConn1
